simulink model "gm_sampleModel1652_sub"  (R2023a)
settings: Solver=VariableStepAuto  StartTime=0.0  StopTime=10.0  RelTol=1e-3
libraries: hdlsllib x3, simulink x2
settings Model: Creator=user1  LastModifiedBy=user1
settings OptimizationCC: BlockReduction=off  ConditionallyExecuteInputs=off
settings DebuggingCC: InheritedTsInSrcMsg=none

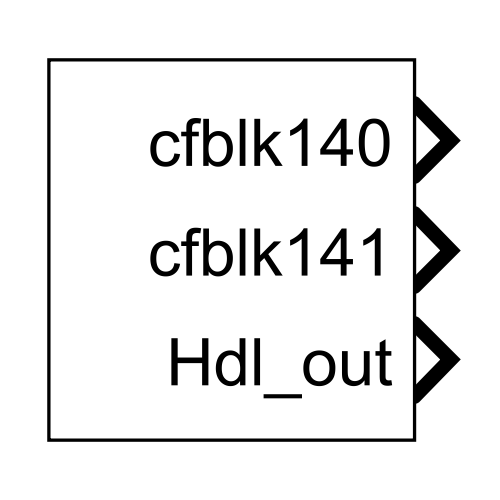
[thumbnail: Simulink's stored preview of the top-level diagram]
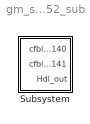
== system gm_sampleModel1652_sub ==
  Subsystem : Subsystem

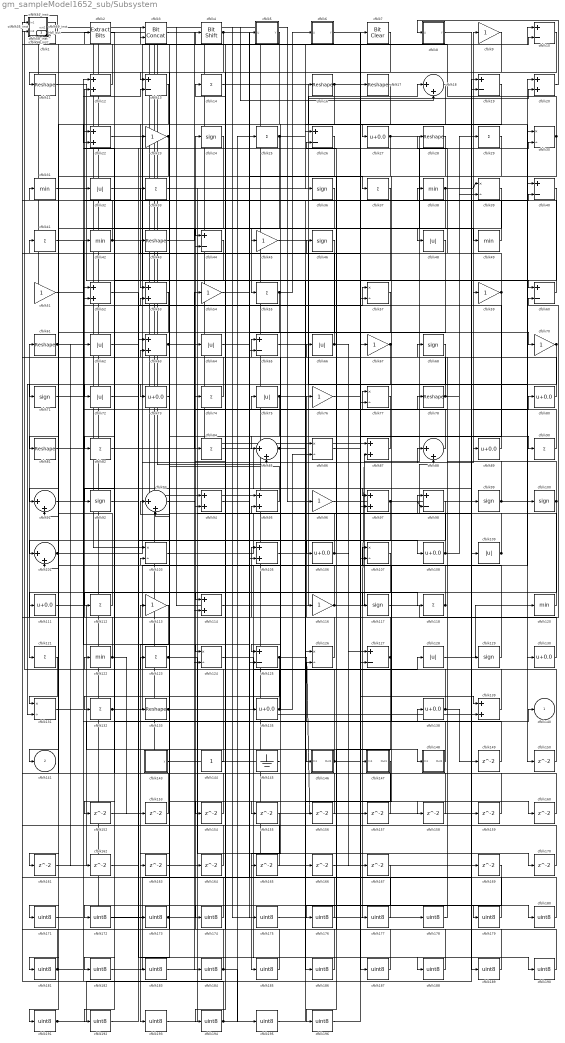
== system gm_sampleModel1652_sub/Subsystem ==
  cfblk1 : hdlsllib/Logic and Bit Operations/Bit Slice  lidx=7  ridx=0
  cfblk{10,13,19,26,40,44,60,65,98,125,127} (11 alike) : Sum  Inputs=+-  OutDataTypeStr=uint8
  cfblk{24,36,46,68,71,92,99..100,117,129} (10 alike) : Signum
  cfblk{18,85,88,91,93,101} (6 alike) : Sum  Inputs=|++  OutDataTypeStr=uint8
  cfblk102_inst : Subsystem
  cfblk{30,39,57,77,86,103,107,124,126,131} (10 alike) : Product  Inputs=*/  OutDataTypeStr=uint8  RndMeth=Zero  SaturateOnIntegerOverflow=on
  cfblk104_inst : Subsystem
  cfblk{12,20,22,52..53,63,87,94..95,97,105,114,139} (13 alike) : Sum  OutDataTypeStr=uint8
  cfblk{27,73,80,89,106,108,111,130,135,138} (10 alike) : Bias  Bias=0.0  SaturateOnIntegerOverflow=off
  cfblk{32,48,62,64,66,72,75,109,128} (9 alike) : Abs  OutDataTypeStr=uint8  SaturateOnIntegerOverflow=off
  cfblk{11,16..17,28,43,61,78,81,133} (9 alike) : Reshape
  cfblk{14,25,29,33,37,41,55,74,82,84,90,112,118,121,123,132} (16 alike) : Sum  Inputs=+  OutDataTypeStr=uint8
  cfblk{9,23,45,51,54,59,67,70,76,96,113,116} (12 alike) : Gain  OutDataTypeStr=uint8
  cfblk119_inst : Subsystem
  cfblk{31,38,42,49,120,122} (6 alike) : MinMax  OutDataTypeStr=uint8
  cfblk143 : Subsystem  mask(Counter Limited){uplimit=double(7), tsamp=double(-1)}
      mask prompts: uplimit "Simulink:masks:UpperLimit_MP"; tsamp "Simulink:masks:SampleTime_MP"
      mask help: Simulink:masks:CounterLimited_MD
      mask init:
      | nbits = double(8);
      | tsamp = double(-1);
      | uplimit = double(7);
  cfblk144 : Constant  OutDataTypeStr=uint8  SampleTime=-1
  cfblk145 : Ground
  cfblk146 : Subsystem
  cfblk147 : Subsystem
  cfblk148 : Subsystem
  cfblk{149..150,152..167,169..170} (20 alike) : Delay  SampleTime=1
  cfblk15_inst : Subsystem
  cfblk{171..196} (26 alike) : DataTypeConversion  OutDataTypeStr=uint8  SaturateOnIntegerOverflow=off  RndMeth=Floor
  cfblk2 : simulink/Logic and Bit Operations/Extract Bits  bitsToExtract=Upper half  numBits=8  bitIdxRange=[0 7]  outScalingMode=Preserve fixed-point scaling
      settings: LibrarySourceBlock=|
      | hdlsllib/Logic and Bit
      | Operations/Extract Bits
  cfblk21_inst : Subsystem
  cfblk3 : hdlsllib/Logic and Bit Operations/Bit Concat  numInputs=2
  cfblk34_inst : Subsystem
  cfblk35_inst : Subsystem
  cfblk4 : hdlsllib/Logic and Bit Operations/Bit Shift  mode=Shift Left Logical  N=0
  cfblk5 : Subsystem  mask(Detect Rise Positive){vinit=double(0), InputProcessing=Elements as channels (sample based), OutDataTypeStr=uint8}
      mask prompts: vinit "Simulink:masks:InitialCondition_MP"; InputProcessing "Simulink:masks:InputProcessing_MP"; OutDataTypeStr "Simulink:masks:OutputDataType_MP"
      mask help: Simulink:masks:DetectRisePositive_MD
      mask init:
      | InputProcessing = 'Elements as channels (sample based)';
      | OutDataTypeStr = 'uint8';
      | vinit = double(0);
      mask TypeOptions InputProcessing: Simulink:masks:ColumnsAsChannelsFrameBased | Simulink:masks:ElementsAsChannelsSampleBased
      mask TypeOptions OutDataTypeStr: Simulink:masks:uint8 | Simulink:masks:boolean
      mask Display: fprintf('U > 0\n&  NOT\nU/z > 0')
  cfblk56_inst : Subsystem
  cfblk58_inst : Subsystem
  cfblk6 : Subsystem  mask(Detect Rise Positive){vinit=double(0), InputProcessing=Elements as channels (sample based), OutDataTypeStr=uint8}
      mask prompts: vinit "Simulink:masks:InitialCondition_MP"; InputProcessing "Simulink:masks:InputProcessing_MP"; OutDataTypeStr "Simulink:masks:OutputDataType_MP"
      mask help: Simulink:masks:DetectRisePositive_MD
      mask init:
      | InputProcessing = 'Elements as channels (sample based)';
      | OutDataTypeStr = 'uint8';
      | vinit = double(0);
      mask TypeOptions InputProcessing: Simulink:masks:ColumnsAsChannelsFrameBased | Simulink:masks:ElementsAsChannelsSampleBased
      mask TypeOptions OutDataTypeStr: Simulink:masks:uint8 | Simulink:masks:boolean
      mask Display: fprintf('U > 0\n&  NOT\nU/z > 0')
  cfblk69_inst : Subsystem
  cfblk7 : simulink/Logic and Bit Operations/Bit Clear  iBit=0
      settings: LibrarySourceBlock=|
      | hdlsllib/Logic and Bit
      | Operations/Bit Clear
  cfblk8 : Subsystem  mask(Detect Fall Negative){vinit=double(0), InputProcessing=Elements as channels (sample based), OutDataTypeStr=uint8}
      mask prompts: vinit "Simulink:masks:InitialCondition_MP"; InputProcessing "Simulink:masks:InputProcessing_MP"; OutDataTypeStr "Simulink:masks:OutputDataType_MP"
      mask help: Simulink:masks:DetectFallNegative_MD
      mask init:
      | InputProcessing = 'Elements as channels (sample based)';
      | OutDataTypeStr = 'uint8';
      | vinit = double(0);
      mask TypeOptions InputProcessing: Simulink:masks:ColumnsAsChannelsFrameBased | Simulink:masks:ElementsAsChannelsSampleBased
      mask TypeOptions OutDataTypeStr: Simulink:masks:uint8 | Simulink:masks:boolean
      mask Display: fprintf('U < 0\n&  NOT\nU/z < 0')
  cfblk140 : Outport  OutDataTypeStr=uint8  SampleTime=1  VectorParamsAs1DForOutWhenUnconnected=off
  cfblk141 : Outport  Port=2  OutDataTypeStr=uint8  SampleTime=1  VectorParamsAs1DForOutWhenUnconnected=off
  Hdl_out : Outport  Port=3  OutDataTypeStr=uint8  SampleTime=1
  wires:
  cfblk1/1 -> cfblk104_inst/1(in1)
  cfblk10/1 -> cfblk11/1
  cfblk100/1 -> cfblk177/1, cfblk9/1
  cfblk101/1 -> cfblk89/1, cfblk10/2
  cfblk102_inst/1(out1) -> cfblk95/1, cfblk87/1
  cfblk103/1 -> cfblk88/2
  cfblk104_inst/1(out1) -> cfblk103/1
  cfblk105/1 -> cfblk18/1
  cfblk106/1 -> cfblk56_inst/1(in1), cfblk127/1
  cfblk107/1 -> cfblk121/1
  cfblk108/1 -> cfblk65/1, cfblk39/2
  cfblk109/1 -> cfblk98/1, cfblk41/1
  cfblk11/1 -> cfblk60/1
  cfblk111/1 -> cfblk147/1(In1)
  cfblk112/1 -> cfblk15_inst/1(in1)
  cfblk113/1 -> cfblk193/1
  cfblk114/1 -> cfblk20/2
  cfblk116/1 -> cfblk87/2, cfblk12/2, cfblk30/2
  cfblk117/1 -> cfblk60/2
  cfblk118/1 -> cfblk21_inst/1(in1), cfblk42/1
  cfblk119_inst/1(out1) -> cfblk100/1
  cfblk12/1 -> cfblk102_inst/1(in1)
  cfblk120/1 -> cfblk78/1
  cfblk121/1 -> cfblk131/1
  cfblk122/1 -> cfblk69_inst/1(in1), cfblk153/1
  cfblk123/1 -> cfblk36/1, cfblk170/1
  cfblk124/1 -> cfblk190/1
  cfblk125/1 -> cfblk156/1, cfblk132/1
  cfblk126/1 -> cfblk52/1
  cfblk127/1 -> cfblk176/1, cfblk105/1, cfblk76/1
  cfblk128/1 -> cfblk120/1
  cfblk129/1 -> cfblk62/1
  cfblk13/1 -> cfblk172/1
  cfblk130/1 -> cfblk61/1
  cfblk131/1 -> cfblk13/2
  cfblk132/1 -> cfblk24/1, cfblk67/1
  cfblk133/1 -> cfblk20/1, cfblk17/1, cfblk128/1
  cfblk135/1 -> cfblk95/2, cfblk22/1, cfblk86/2
  cfblk138/1 -> cfblk26/2, cfblk149/1
  cfblk139/1 -> cfblk4/1
  cfblk14/1 -> cfblk150/1
  cfblk143/1(y) -> cfblk53/2
  cfblk144/1 -> cfblk35_inst/2(in2)
  cfblk145/1 -> cfblk1/1
  cfblk146/1(Out1) -> cfblk140/1, cfblk123/1
  cfblk147/1(Out1) -> cfblk163/1
  cfblk148/1(Out1) -> cfblk122/1
  cfblk149/1 -> cfblk107/1
  cfblk15_inst/1(out1) -> cfblk159/1
  cfblk150/1 -> cfblk103/2
  cfblk152/1 -> cfblk40/2
  cfblk153/1 -> cfblk119_inst/2(in2)
  cfblk154/1 -> cfblk91/2
  cfblk155/1 -> cfblk185/1
  cfblk156/1 -> cfblk63/2
  cfblk157/1 -> cfblk21_inst/2(in2)
  cfblk158/1 -> cfblk52/2
  cfblk159/1 -> cfblk101/2
  cfblk16/1 -> cfblk125/1, cfblk90/1
  cfblk160/1 -> cfblk104_inst/2(in2)
  cfblk161/1 -> cfblk126/2
  cfblk162/1 -> cfblk30/1
  cfblk163/1 -> cfblk88/1
  cfblk164/1 -> cfblk58_inst/2(in2)
  cfblk165/1 -> cfblk44/2
  cfblk166/1 -> cfblk97/2
  cfblk167/1 -> cfblk182/1
  cfblk169/1 -> cfblk196/1
  cfblk17/1 -> cfblk53/1
  cfblk170/1 -> cfblk93/1
  cfblk171/1 -> cfblk138/1
  cfblk172/1 -> cfblk5/1(U)
  cfblk173/1 -> cfblk7/1, Hdl_out/1
  cfblk174/1 -> cfblk64/1
  cfblk175/1 -> cfblk180/1
  cfblk176/1 -> cfblk94/1
  cfblk177/1 -> cfblk94/2
  cfblk178/1 -> cfblk68/1
  cfblk179/1 -> cfblk34_inst/1(in1)
  cfblk18/1 -> cfblk22/2
  cfblk180/1 -> cfblk34_inst/2(in2)
  cfblk181/1 -> cfblk35_inst/1(in1), cfblk26/1
  cfblk182/1 -> cfblk19/1
  cfblk183/1 -> cfblk19/2
  cfblk184/1 -> cfblk195/1, cfblk113/1
  cfblk185/1 -> cfblk3/1
  cfblk186/1 -> cfblk3/2
  cfblk187/1 -> cfblk119_inst/1(in1)
  cfblk188/1 -> cfblk96/1
  cfblk189/1 -> cfblk164/1
  cfblk19/1 -> cfblk181/1
  cfblk190/1 -> cfblk84/1
  cfblk191/1 -> cfblk99/1, cfblk86/1
  cfblk192/1 -> cfblk57/1
  cfblk193/1 -> cfblk57/2
  cfblk194/1 -> cfblk15_inst/2(in2), cfblk12/1, cfblk25/1
  cfblk195/1 -> cfblk77/1
  cfblk196/1 -> cfblk77/2
  cfblk2/1 -> cfblk82/1
  cfblk20/1 -> cfblk8/1(U)
  cfblk21_inst/1(out1) -> cfblk116/1
  cfblk22/1 -> cfblk48/1
  cfblk23/1 -> cfblk81/1, cfblk192/1
  cfblk24/1 -> cfblk141/1
  cfblk25/1 -> cfblk65/2, cfblk27/1, cfblk10/1
  cfblk26/1 -> cfblk71/1
  cfblk27/1 -> cfblk105/2, cfblk49/1
  cfblk28/1 -> cfblk157/1
  cfblk29/1 -> cfblk114/1
  cfblk3/1 -> cfblk184/1
  cfblk30/1 -> cfblk2/1, cfblk106/1
  cfblk31/1 -> cfblk109/1
  cfblk32/1 -> cfblk186/1
  cfblk33/1 -> cfblk16/1
  cfblk34_inst/1(out1) -> cfblk178/1
  cfblk35_inst/1(out1) -> cfblk139/2, cfblk23/1
  cfblk36/1 -> cfblk44/1
  cfblk37/1 -> cfblk173/1
  cfblk38/1 -> cfblk39/1, cfblk161/1
  cfblk39/1 -> cfblk55/1
  cfblk4/1 -> cfblk13/1, cfblk37/1
  cfblk40/1 -> cfblk92/1
  cfblk41/1 -> cfblk124/1
  cfblk42/1 -> cfblk166/1, cfblk31/1
  cfblk43/1 -> cfblk45/1
  cfblk44/1 -> cfblk72/1
  cfblk45/1 -> cfblk130/1
  cfblk46/1 -> cfblk91/1
  cfblk48/1 -> cfblk152/1
  cfblk49/1 -> cfblk58_inst/1(in1)
  cfblk5/1(Y) -> cfblk171/1
  cfblk51/1 -> cfblk40/1
  cfblk52/1 -> cfblk188/1
  cfblk53/1 -> cfblk111/1
  cfblk54/1 -> cfblk135/1
  cfblk55/1 -> cfblk73/1, cfblk6/1(U)
  cfblk56_inst/1(out1) -> cfblk85/2
  cfblk57/1 -> cfblk191/1
  cfblk58_inst/1(out1) -> cfblk51/1, cfblk169/1
  cfblk59/1 -> cfblk56_inst/2(in2), cfblk28/1, cfblk127/2
  cfblk6/1(Y) -> cfblk179/1
  cfblk60/1 -> cfblk14/1
  cfblk61/1 -> cfblk125/2, cfblk162/1
  cfblk62/1 -> cfblk148/1(In1)
  cfblk63/1 -> cfblk124/2, cfblk118/1
  cfblk64/1 -> cfblk70/1
  cfblk65/1 -> cfblk126/1
  cfblk66/1 -> cfblk69_inst/2(in2), cfblk167/1
  cfblk67/1 -> cfblk155/1, cfblk131/2
  cfblk68/1 -> cfblk112/1
  cfblk69_inst/1(out1) -> cfblk18/2
  cfblk7/1 -> cfblk174/1
  cfblk70/1 -> cfblk114/2, cfblk154/1
  cfblk71/1 -> cfblk117/1
  cfblk72/1 -> cfblk46/1
  cfblk73/1 -> cfblk133/1
  cfblk74/1 -> cfblk63/1
  cfblk75/1 -> cfblk93/2, cfblk107/2
  cfblk76/1 -> cfblk158/1
  cfblk77/1 -> cfblk194/1
  cfblk78/1 -> cfblk43/1, cfblk29/1
  cfblk8/1(Y) -> cfblk129/1
  cfblk80/1 -> cfblk102_inst/2(in2)
  cfblk81/1 -> cfblk80/1
  cfblk82/1 -> cfblk54/1
  cfblk84/1 -> cfblk189/1
  cfblk85/1 -> cfblk160/1, cfblk38/1
  cfblk86/1 -> cfblk139/1
  cfblk87/1 -> cfblk85/1
  cfblk88/1 -> cfblk75/1
  cfblk89/1 -> cfblk32/1
  cfblk9/1 -> cfblk183/1
  cfblk90/1 -> cfblk59/1
  cfblk91/1 -> cfblk97/1
  cfblk92/1 -> cfblk108/1
  cfblk93/1 -> cfblk146/1(In1)
  cfblk94/1 -> cfblk175/1
  cfblk95/1 -> cfblk33/1
  cfblk96/1 -> cfblk187/1
  cfblk97/1 -> cfblk98/2, cfblk101/1
  cfblk98/1 -> cfblk165/1
  cfblk99/1 -> cfblk66/1, cfblk74/1

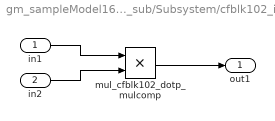
== system gm_sampleModel1652_sub/Subsystem/cfblk102_inst ==
  in1 : Inport  OutDataTypeStr=uint8  SampleTime=1
  in2 : Inport  Port=2  OutDataTypeStr=uint8  SampleTime=1
  mul_cfblk102_dotp_mulcomp : Product  Inputs=**  OutDataTypeStr=uint8  SampleTime=1
  out1 : Outport  OutDataTypeStr=uint8  SampleTime=1
  wires:
  in1/1 -> mul_cfblk102_dotp_mulcomp/1
  in2/1 -> mul_cfblk102_dotp_mulcomp/2
  mul_cfblk102_dotp_mulcomp/1 -> out1/1

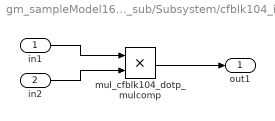
== system gm_sampleModel1652_sub/Subsystem/cfblk104_inst ==
  in1 : Inport  OutDataTypeStr=uint8  SampleTime=1
  in2 : Inport  Port=2  OutDataTypeStr=uint8  SampleTime=1
  mul_cfblk104_dotp_mulcomp : Product  Inputs=**  OutDataTypeStr=uint8  SampleTime=1
  out1 : Outport  OutDataTypeStr=uint8  SampleTime=1
  wires:
  in1/1 -> mul_cfblk104_dotp_mulcomp/1
  in2/1 -> mul_cfblk104_dotp_mulcomp/2
  mul_cfblk104_dotp_mulcomp/1 -> out1/1

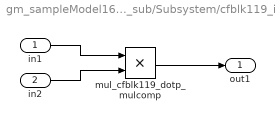
== system gm_sampleModel1652_sub/Subsystem/cfblk119_inst ==
  in1 : Inport  OutDataTypeStr=uint8  SampleTime=1
  in2 : Inport  Port=2  OutDataTypeStr=uint8  SampleTime=1
  mul_cfblk119_dotp_mulcomp : Product  Inputs=**  OutDataTypeStr=uint8  SampleTime=1
  out1 : Outport  OutDataTypeStr=uint8  SampleTime=1
  wires:
  in1/1 -> mul_cfblk119_dotp_mulcomp/1
  in2/1 -> mul_cfblk119_dotp_mulcomp/2
  mul_cfblk119_dotp_mulcomp/1 -> out1/1

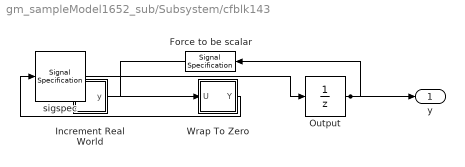
== system gm_sampleModel1652_sub/Subsystem/cfblk143 ==
  Force to be scalar : SignalSpecification  DisableCoverage=on  Dimensions=1
  Increment Real World : Subsystem  mask(Real World Value Increment){}
      mask help: Simulink:masks:RealWorldValueIncrement_MD
      mask Display: disp('V++')
  Output : UnitDelay  InitialCondition=0.0  SampleTime=tsamp  HasFrameUpgradeWarning=on
  Wrap To Zero : Subsystem  mask(Wrap To Zero){Threshold=double(7)}
      mask prompts: Threshold "Simulink:masks:Threshold_MP"
      mask help: Simulink:masks:WrapToZero_MD
  sigspec : SignalSpecification  OutDataTypeStr=uint8  Dimensions=1
  y : Outport  SampleTime=1
  wires:
  Force to be scalar/1 -> Increment Real World/1(u)
  Increment Real World/1(y) -> Wrap To Zero/1(U)
  Output/1 -> Force to be scalar/1, y/1
  Wrap To Zero/1(Y) -> sigspec/1
  sigspec/1 -> Output/1

== system gm_sampleModel1652_sub/Subsystem/cfblk146 ==
  In1 : Inport  OutDataTypeStr=uint8  PortDimensions=1  SampleTime=1
  Out1 : Outport  SampleTime=1
  wires:
  In1/1 -> Out1/1

== system gm_sampleModel1652_sub/Subsystem/cfblk147 ==
  In1 : Inport  OutDataTypeStr=uint8  PortDimensions=1  SampleTime=1
  Out1 : Outport  SampleTime=1
  wires:
  In1/1 -> Out1/1

== system gm_sampleModel1652_sub/Subsystem/cfblk148 ==
  In1 : Inport  OutDataTypeStr=uint8  PortDimensions=1  SampleTime=1
  Out1 : Outport  SampleTime=1
  wires:
  In1/1 -> Out1/1

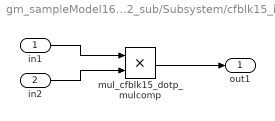
== system gm_sampleModel1652_sub/Subsystem/cfblk15_inst ==
  in1 : Inport  OutDataTypeStr=uint8  SampleTime=1
  in2 : Inport  Port=2  OutDataTypeStr=uint8  SampleTime=1
  mul_cfblk15_dotp_mulcomp : Product  Inputs=**  OutDataTypeStr=uint8  SampleTime=1
  out1 : Outport  OutDataTypeStr=uint8  SampleTime=1
  wires:
  in1/1 -> mul_cfblk15_dotp_mulcomp/1
  in2/1 -> mul_cfblk15_dotp_mulcomp/2
  mul_cfblk15_dotp_mulcomp/1 -> out1/1

== system gm_sampleModel1652_sub/Subsystem/cfblk21_inst ==
  in1 : Inport  OutDataTypeStr=uint8  SampleTime=1
  in2 : Inport  Port=2  OutDataTypeStr=uint8  SampleTime=1
  mul_cfblk21_dotp_mulcomp : Product  Inputs=**  OutDataTypeStr=uint8  SampleTime=1
  out1 : Outport  OutDataTypeStr=uint8  SampleTime=1
  wires:
  in1/1 -> mul_cfblk21_dotp_mulcomp/1
  in2/1 -> mul_cfblk21_dotp_mulcomp/2
  mul_cfblk21_dotp_mulcomp/1 -> out1/1

== system gm_sampleModel1652_sub/Subsystem/cfblk34_inst ==
  in1 : Inport  OutDataTypeStr=uint8  SampleTime=1
  in2 : Inport  Port=2  OutDataTypeStr=uint8  SampleTime=1
  mul_cfblk34_dotp_mulcomp : Product  Inputs=**  OutDataTypeStr=uint8  SampleTime=1
  out1 : Outport  OutDataTypeStr=uint8  SampleTime=1
  wires:
  in1/1 -> mul_cfblk34_dotp_mulcomp/1
  in2/1 -> mul_cfblk34_dotp_mulcomp/2
  mul_cfblk34_dotp_mulcomp/1 -> out1/1

== system gm_sampleModel1652_sub/Subsystem/cfblk35_inst ==
  in1 : Inport  OutDataTypeStr=uint8  SampleTime=1
  in2 : Inport  Port=2  OutDataTypeStr=uint8  SampleTime=1
  mul_cfblk35_dotp_mulcomp : Product  Inputs=**  OutDataTypeStr=uint8  SampleTime=1
  out1 : Outport  OutDataTypeStr=uint8  SampleTime=1
  wires:
  in1/1 -> mul_cfblk35_dotp_mulcomp/1
  in2/1 -> mul_cfblk35_dotp_mulcomp/2
  mul_cfblk35_dotp_mulcomp/1 -> out1/1

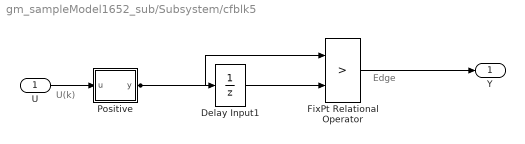
== system gm_sampleModel1652_sub/Subsystem/cfblk5 ==
  note: U(k)
  note: Edge
  U : Inport  OutDataTypeStr=uint8  SampleTime=1
  Delay Input1 : UnitDelay  Description=Store in Global RAM  DisableCoverage=on  InitialCondition=vinit  SampleTime=-1  HasFrameUpgradeWarning=on
  FixPt Relational Operator : RelationalOperator  Operator=>  OutDataTypeStr=fixdt(0, 8)  ZeroCross=off  InputSameDT=off
  Positive : Subsystem  mask(Compare To Zero){relop=>, OutDataTypeStr=boolean, ZeroCross=off}
      mask prompts: relop "Simulink:masks:Operator_MP"; OutDataTypeStr "Simulink:masks:OutputDataType_MP"; ZeroCross "Simulink:masks:EnableZerocrossingDetection_MP"
      mask help: Simulink:masks:CompareToZero_MD
      mask init:
      | OutDataTypeStr = 'boolean';
      | ZeroCross = 'off';
      | blkName = 'sampleModel1652_sub/Subsystem/cfblk5/Positive';
      | relop = '>';
      | setValue = 'boolean';
      mask TypeOptions relop: == | ~= | < | <= | >= | >
      mask TypeOptions OutDataTypeStr: Simulink:masks:uint8 | Simulink:masks:boolean
      mask Callback ZeroCross: sl('zeroCrossEnable', gcbh);
      mask Display: disp([relop,' 0'])
  Y : Outport  SampleTime=1
  wires:
  U/1 -> Positive/1(u)
  Delay Input1/1 -> FixPt Relational Operator/2
  FixPt Relational Operator/1 -> Y/1
  Positive/1(y) -> FixPt Relational Operator/1, Delay Input1/1

== system gm_sampleModel1652_sub/Subsystem/cfblk56_inst ==
  in1 : Inport  OutDataTypeStr=uint8  SampleTime=1
  in2 : Inport  Port=2  OutDataTypeStr=uint8  SampleTime=1
  mul_cfblk56_dotp_mulcomp : Product  Inputs=**  OutDataTypeStr=uint8  SampleTime=1
  out1 : Outport  OutDataTypeStr=uint8  SampleTime=1
  wires:
  in1/1 -> mul_cfblk56_dotp_mulcomp/1
  in2/1 -> mul_cfblk56_dotp_mulcomp/2
  mul_cfblk56_dotp_mulcomp/1 -> out1/1

== system gm_sampleModel1652_sub/Subsystem/cfblk58_inst ==
  in1 : Inport  OutDataTypeStr=uint8  SampleTime=1
  in2 : Inport  Port=2  OutDataTypeStr=uint8  SampleTime=1
  mul_cfblk58_dotp_mulcomp : Product  Inputs=**  OutDataTypeStr=uint8  SampleTime=1
  out1 : Outport  OutDataTypeStr=uint8  SampleTime=1
  wires:
  in1/1 -> mul_cfblk58_dotp_mulcomp/1
  in2/1 -> mul_cfblk58_dotp_mulcomp/2
  mul_cfblk58_dotp_mulcomp/1 -> out1/1

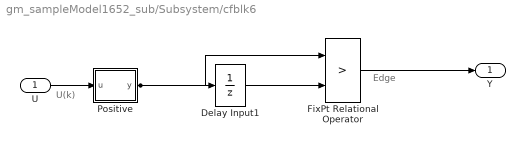
== system gm_sampleModel1652_sub/Subsystem/cfblk6 ==
  note: U(k)
  note: Edge
  U : Inport  OutDataTypeStr=uint8  SampleTime=1
  Delay Input1 : UnitDelay  Description=Store in Global RAM  DisableCoverage=on  InitialCondition=vinit  SampleTime=-1  HasFrameUpgradeWarning=on
  FixPt Relational Operator : RelationalOperator  Operator=>  OutDataTypeStr=fixdt(0, 8)  ZeroCross=off  InputSameDT=off
  Positive : Subsystem  mask(Compare To Zero){relop=>, OutDataTypeStr=boolean, ZeroCross=off}
      mask prompts: relop "Simulink:masks:Operator_MP"; OutDataTypeStr "Simulink:masks:OutputDataType_MP"; ZeroCross "Simulink:masks:EnableZerocrossingDetection_MP"
      mask help: Simulink:masks:CompareToZero_MD
      mask init:
      | OutDataTypeStr = 'boolean';
      | ZeroCross = 'off';
      | blkName = 'sampleModel1652_sub/Subsystem/cfblk6/Positive';
      | relop = '>';
      | setValue = 'boolean';
      mask TypeOptions relop: == | ~= | < | <= | >= | >
      mask TypeOptions OutDataTypeStr: Simulink:masks:uint8 | Simulink:masks:boolean
      mask Callback ZeroCross: sl('zeroCrossEnable', gcbh);
      mask Display: disp([relop,' 0'])
  Y : Outport  SampleTime=1
  wires:
  U/1 -> Positive/1(u)
  Delay Input1/1 -> FixPt Relational Operator/2
  FixPt Relational Operator/1 -> Y/1
  Positive/1(y) -> FixPt Relational Operator/1, Delay Input1/1

== system gm_sampleModel1652_sub/Subsystem/cfblk69_inst ==
  in1 : Inport  OutDataTypeStr=uint8  SampleTime=1
  in2 : Inport  Port=2  OutDataTypeStr=uint8  SampleTime=1
  mul_cfblk69_dotp_mulcomp : Product  Inputs=**  OutDataTypeStr=uint8  SampleTime=1
  out1 : Outport  OutDataTypeStr=uint8  SampleTime=1
  wires:
  in1/1 -> mul_cfblk69_dotp_mulcomp/1
  in2/1 -> mul_cfblk69_dotp_mulcomp/2
  mul_cfblk69_dotp_mulcomp/1 -> out1/1

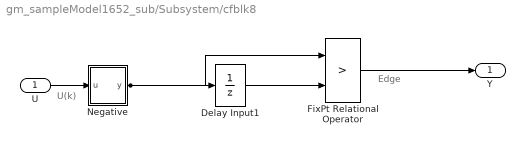
== system gm_sampleModel1652_sub/Subsystem/cfblk8 ==
  note: U(k)
  note: Edge
  U : Inport  OutDataTypeStr=uint8  SampleTime=1
  Delay Input1 : UnitDelay  Description=Store in Global RAM  DisableCoverage=on  InitialCondition=vinit  SampleTime=-1  HasFrameUpgradeWarning=on
  FixPt Relational Operator : RelationalOperator  Operator=>  OutDataTypeStr=fixdt(0, 8)  ZeroCross=off  InputSameDT=off
  Negative : Subsystem  mask(Compare To Zero){relop=<, OutDataTypeStr=boolean, ZeroCross=off}
      mask prompts: relop "Simulink:masks:Operator_MP"; OutDataTypeStr "Simulink:masks:OutputDataType_MP"; ZeroCross "Simulink:masks:EnableZerocrossingDetection_MP"
      mask help: Simulink:masks:CompareToZero_MD
      mask init:
      | OutDataTypeStr = 'boolean';
      | ZeroCross = 'off';
      | blkName = 'sampleModel1652_sub/Subsystem/cfblk8/Negative';
      | relop = '<';
      | setValue = 'boolean';
      mask TypeOptions relop: == | ~= | < | <= | >= | >
      mask TypeOptions OutDataTypeStr: Simulink:masks:uint8 | Simulink:masks:boolean
      mask Callback ZeroCross: sl('zeroCrossEnable', gcbh);
      mask Display: disp([relop,' 0'])
  Y : Outport  SampleTime=1
  wires:
  U/1 -> Negative/1(u)
  Delay Input1/1 -> FixPt Relational Operator/2
  FixPt Relational Operator/1 -> Y/1
  Negative/1(y) -> FixPt Relational Operator/1, Delay Input1/1

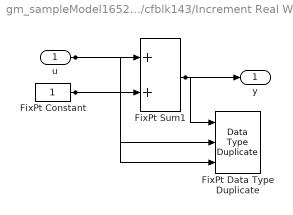
== system gm_sampleModel1652_sub/Subsystem/cfblk143/Increment Real World ==
  u : Inport  OutDataTypeStr=uint8  SampleTime=1
  FixPt Constant : Constant  DisableCoverage=on  OutDataTypeStr=Inherit: Inherit via back propagation  SampleTime=-1
  FixPt Data Type Duplicate : DataTypeDuplicate  DisableCoverage=on  NumInputPorts=3
  FixPt Sum1 : Sum  InputSameDT=on  OutDataTypeStr=Inherit: Inherit via back propagation  LockScale=on
  y : Outport  SampleTime=1
  wires:
  u/1 -> FixPt Sum1/1, FixPt Data Type Duplicate/2
  FixPt Constant/1 -> FixPt Sum1/2, FixPt Data Type Duplicate/3
  FixPt Sum1/1 -> FixPt Data Type Duplicate/1, y/1

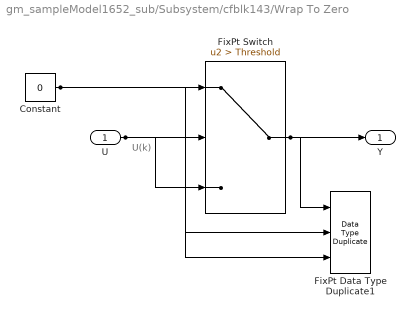
== system gm_sampleModel1652_sub/Subsystem/cfblk143/Wrap To Zero ==
  note: U(k)
  U : Inport  OutDataTypeStr=uint8  SampleTime=1
  Constant : Constant  DisableCoverage=on  Value=0  OutDataTypeStr=Inherit: Inherit via back propagation  SampleTime=-1
  FixPt Data Type Duplicate1 : DataTypeDuplicate  DisableCoverage=on  NumInputPorts=3
  FixPt Switch : Switch  Criteria=u2 > Threshold  Threshold=Threshold  OutDataTypeStr=Inherit: Inherit via back propagation  ZeroCross=off  SaturateOnIntegerOverflow=off  InputSameDT=off
  Y : Outport  SampleTime=1
  wires:
  U/1 -> FixPt Switch/3, FixPt Switch/2, FixPt Data Type Duplicate1/2
  Constant/1 -> FixPt Switch/1, FixPt Data Type Duplicate1/3
  FixPt Switch/1 -> FixPt Data Type Duplicate1/1, Y/1

== system gm_sampleModel1652_sub/Subsystem/cfblk5/Positive ==
  u : Inport  OutDataTypeStr=uint8  SampleTime=1
  Compare : RelationalOperator  Operator=>  OutDataTypeStr=boolean  ZeroCross=off
  Constant : Constant  DisableCoverage=on  Value=0  OutDataTypeStr=Inherit: Inherit via back propagation  SampleTime=-1  PreserveConstantTs=on
  y : Outport  SampleTime=1
  wires:
  u/1 -> Compare/1
  Compare/1 -> y/1
  Constant/1 -> Compare/2

== system gm_sampleModel1652_sub/Subsystem/cfblk6/Positive ==
  u : Inport  OutDataTypeStr=uint8  SampleTime=1
  Compare : RelationalOperator  Operator=>  OutDataTypeStr=boolean  ZeroCross=off
  Constant : Constant  DisableCoverage=on  Value=0  OutDataTypeStr=Inherit: Inherit via back propagation  SampleTime=-1  PreserveConstantTs=on
  y : Outport  SampleTime=1
  wires:
  u/1 -> Compare/1
  Compare/1 -> y/1
  Constant/1 -> Compare/2

== system gm_sampleModel1652_sub/Subsystem/cfblk8/Negative ==
  u : Inport  OutDataTypeStr=uint8  SampleTime=1
  Compare : RelationalOperator  Operator=<  OutDataTypeStr=boolean  ZeroCross=off
  Constant : Constant  DisableCoverage=on  Value=0  OutDataTypeStr=Inherit: Inherit via back propagation  SampleTime=-1  PreserveConstantTs=on
  y : Outport  SampleTime=1
  wires:
  u/1 -> Compare/1
  Compare/1 -> y/1
  Constant/1 -> Compare/2
